simulink subsystem "ControlObject"  (R2022b)
settings: Solver=VariableStepAuto  StartTime=0.0  StopTime=10.0  RelTol=1e-3
model mask{motor_nominal_voltage=0, L=0, R=0, km=0, kw=0, J_motor=0, vis_friction_coef_motor=0, i_gear=0, J_gear=0, vis_friction_coef_gear=0, r_cyl=0, vis_friction_coef_cradle=0, cradle_mass=0}
  mask prompts: motor_nominal_voltage "Motor nominal voltage, V"; L "Rotor inductance, H"; R "Rotor resistance, Ohm"; km "Torque constant"; kw "Speed constant"; J_motor "Motor inertia, kg * m^2"; vis_friction_coef_motor "Viscous friction coefficient, kg * m^2 / s"; i_gear "Gear aspect ratio"; J_gear "Gear inertia, kg * m^2"; vis_friction_coef_gear "Viscous friction coefficient, kg * m^2 / s"; r_cyl "Radius of the working cylinder, m"; vis_friction_coef_cradle "Viscous friction coefficient, kg * m^2 / s"; cradle_mass "Cradle mass, kg"
settings Model: Creator=Ilya_Andriyanov  LastModifiedBy=Ilya_Andriyanov
settings OptimizationCC: ReuseModelBlockBuffer=on

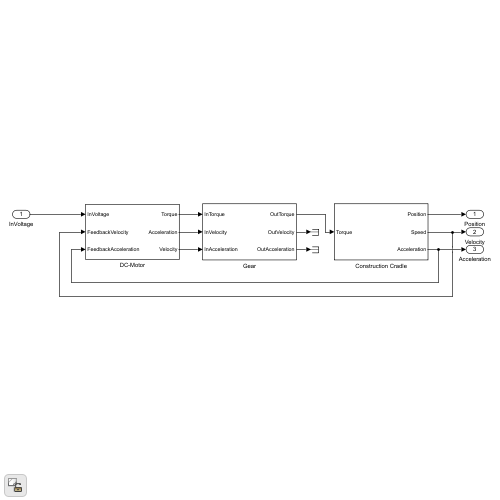
[thumbnail: Simulink's stored preview of the top-level diagram]
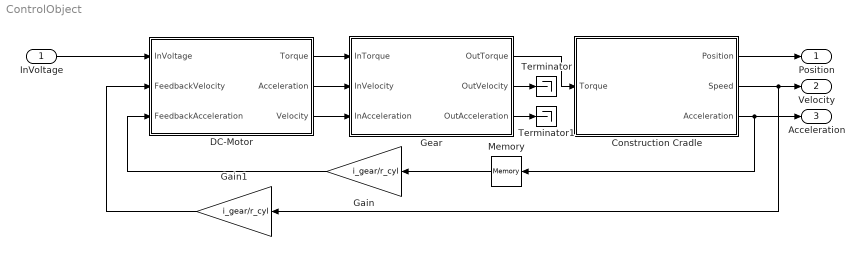
== system ControlObject ==
  InVoltage : Inport
  Construction Cradle : Subsystem
  DC-Motor : Subsystem
  Gain : Gain  Gain=i_gear/r_cyl
  Gain1 : Gain  Gain=i_gear/r_cyl
  Gear : Subsystem
  Memory : Memory
  Terminator : Terminator
  Terminator1 : Terminator
  Position : Outport
  Velocity : Outport  Port=2
  Acceleration : Outport  Port=3
  wires:
  InVoltage/1 -> DC-Motor/1(InVoltage)
  DC-Motor/1(Torque) -> Gear/1(InTorque)
  DC-Motor/2(Acceleration) -> Gear/2(InVelocity)
  DC-Motor/3(Velocity) -> Gear/3(InAcceleration)
  Gear/2(OutVelocity) -> Terminator/1
  Gear/3(OutAcceleration) -> Terminator1/1
  Gear/1(OutTorque) -> Construction Cradle/1(Torque)
  Construction Cradle/1(Position) -> Position/1
  Construction Cradle/2(Speed) -> Gain1/1, Velocity/1
  Construction Cradle/3(Acceleration) -> Memory/1, Acceleration/1
  Memory/1 -> Gain/1
  Gain/1 -> DC-Motor/3(FeedbackAcceleration)
  Gain1/1 -> DC-Motor/2(FeedbackVelocity)

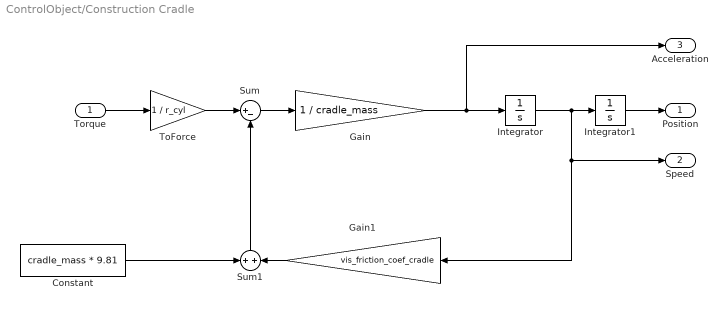
== system ControlObject/Construction Cradle ==
  Torque : Inport
  Constant : Constant  Value=cradle_mass * 9.81
  Gain : Gain  Gain=1 / cradle_mass
  Gain1 : Gain  Gain=vis_friction_coef_cradle
  Integrator : Integrator
  Integrator1 : Integrator
  Sum : Sum  Inputs=|+-
  Sum1 : Sum  Inputs=+|+
  ToForce : Gain  Gain=1 / r_cyl
  Position : Outport
  Speed : Outport  Port=2
  Acceleration : Outport  Port=3
  wires:
  Torque/1 -> ToForce/1
  ToForce/1 -> Sum/1
  Sum/1 -> Gain/1
  Integrator/1 -> Speed/1, Gain1/1, Integrator1/1
  Integrator1/1 -> Position/1
  Constant/1 -> Sum1/1
  Sum1/1 -> Sum/2
  Gain/1 -> Integrator/1, Acceleration/1
  Gain1/1 -> Sum1/2

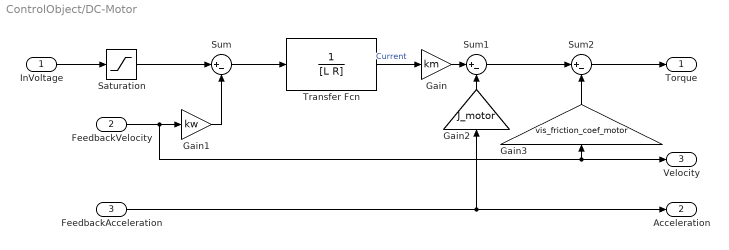
== system ControlObject/DC-Motor ==
  InVoltage : Inport
  FeedbackVelocity : Inport  Port=2
  FeedbackAcceleration : Inport  Port=3
  Gain : Gain  Gain=km
  Gain1 : Gain  Gain=kw
  Gain2 : Gain  Gain=J_motor
  Gain3 : Gain  Gain=vis_friction_coef_motor
  Saturation : Saturate  UpperLimit=motor_nominal_voltage  LowerLimit=-motor_nominal_voltage
  Sum : Sum  Inputs=|+-
  Sum1 : Sum  Inputs=|+-
  Sum2 : Sum  Inputs=|+-
  Transfer Fcn : TransferFcn  Denominator=[L R]
  Torque : Outport
  Acceleration : Outport  Port=2
  Velocity : Outport  Port=3
  wires:
  Saturation/1 -> Sum/1
  InVoltage/1 -> Saturation/1
  Sum/1 -> Transfer Fcn/1
  Transfer Fcn/1 -> Gain/1  "Current"
  FeedbackVelocity/1 -> Gain3/1, Velocity/1, Gain1/1
  Gain1/1 -> Sum/2
  FeedbackAcceleration/1 -> Acceleration/1, Gain2/1
  Gain/1 -> Sum1/1
  Gain2/1 -> Sum1/2
  Sum1/1 -> Sum2/1
  Sum2/1 -> Torque/1
  Gain3/1 -> Sum2/2

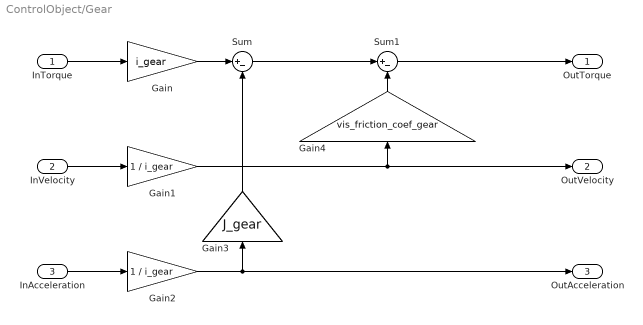
== system ControlObject/Gear ==
  InTorque : Inport
  InVelocity : Inport  Port=2
  InAcceleration : Inport  Port=3
  Gain : Gain  Gain=i_gear
  Gain1 : Gain  Gain=1 / i_gear
  Gain2 : Gain  Gain=1 / i_gear
  Gain3 : Gain  Gain=J_gear
  Gain4 : Gain  Gain=vis_friction_coef_gear
  Sum : Sum  Inputs=|+-
  Sum1 : Sum  Inputs=|+-
  OutTorque : Outport
  OutVelocity : Outport  Port=2
  OutAcceleration : Outport  Port=3
  wires:
  InTorque/1 -> Gain/1
  InVelocity/1 -> Gain1/1
  InAcceleration/1 -> Gain2/1
  Gain2/1 -> Gain3/1, OutAcceleration/1
  Gain1/1 -> Gain4/1, OutVelocity/1
  Gain/1 -> Sum/1
  Sum/1 -> Sum1/1
  Sum1/1 -> OutTorque/1
  Gain3/1 -> Sum/2
  Gain4/1 -> Sum1/2
